simulink model "mainController19a"  (R2019a)
settings: Solver=ode3  StartTime=0  StopTime=inf  FixedStep=0.1  RelTol=1e-3
model workspace (MAT data in the model file):
  SL_ROS_VariableLengthArrays_MaxSizes.CommonInfo.ArrayTruncateAction = 'EmitWarning'
  SL_ROS_VariableLengthArrays_MaxSizes.MsgTypeMap = containers.Map
  SL_ROS_VariableLengthArrays_MaxSizes.MsgTypeMap.serialization.keys = {'sensor_msgs/JointState', 'sensor_msgs/PointCloud2', 'trajectory_msgs/JointTrajectoryPoint'}
  SL_ROS_VariableLengthArrays_MaxSizes.MsgTypeMap.serialization.values{1}(1).PropertyName = 'Name'
  SL_ROS_VariableLengthArrays_MaxSizes.MsgTypeMap.serialization.values{1}(1).DataType = 'std_msgs/String'
  SL_ROS_VariableLengthArrays_MaxSizes.MsgTypeMap.serialization.values{1}(1).MaxLength = 16
  SL_ROS_VariableLengthArrays_MaxSizes.MsgTypeMap.serialization.values{1}(2).PropertyName = 'Position'
  SL_ROS_VariableLengthArrays_MaxSizes.MsgTypeMap.serialization.values{1}(2).DataType = 'double'
  SL_ROS_VariableLengthArrays_MaxSizes.MsgTypeMap.serialization.values{1}(2).MaxLength = 16
  SL_ROS_VariableLengthArrays_MaxSizes.MsgTypeMap.serialization.values{1}(3).PropertyName = 'Velocity'
  SL_ROS_VariableLengthArrays_MaxSizes.MsgTypeMap.serialization.values{1}(3).DataType = 'double'
  SL_ROS_VariableLengthArrays_MaxSizes.MsgTypeMap.serialization.values{1}(3).MaxLength = 16
  SL_ROS_VariableLengthArrays_MaxSizes.MsgTypeMap.serialization.values{1}(4).PropertyName = 'Effort'
  SL_ROS_VariableLengthArrays_MaxSizes.MsgTypeMap.serialization.values{1}(4).DataType = 'double'
  SL_ROS_VariableLengthArrays_MaxSizes.MsgTypeMap.serialization.values{1}(4).MaxLength = 16
  SL_ROS_VariableLengthArrays_MaxSizes.MsgTypeMap.serialization.values{2}(1).PropertyName = 'Data'
  SL_ROS_VariableLengthArrays_MaxSizes.MsgTypeMap.serialization.values{2}(1).DataType = 'uint8'
  SL_ROS_VariableLengthArrays_MaxSizes.MsgTypeMap.serialization.values{2}(1).MaxLength = 9830400
  SL_ROS_VariableLengthArrays_MaxSizes.MsgTypeMap.serialization.values{2}(2).PropertyName = 'Fields'
  SL_ROS_VariableLengthArrays_MaxSizes.MsgTypeMap.serialization.values{2}(2).DataType = 'sensor_msgs/PointField'
  SL_ROS_VariableLengthArrays_MaxSizes.MsgTypeMap.serialization.values{2}(2).MaxLength = 16
  SL_ROS_VariableLengthArrays_MaxSizes.MsgTypeMap.serialization.values{3}(1).PropertyName = 'Positions'
  SL_ROS_VariableLengthArrays_MaxSizes.MsgTypeMap.serialization.values{3}(1).DataType = 'double'
  SL_ROS_VariableLengthArrays_MaxSizes.MsgTypeMap.serialization.values{3}(1).MaxLength = 16
  SL_ROS_VariableLengthArrays_MaxSizes.MsgTypeMap.serialization.values{3}(2).PropertyName = 'Velocities'
  SL_ROS_VariableLengthArrays_MaxSizes.MsgTypeMap.serialization.values{3}(2).DataType = 'double'
  SL_ROS_VariableLengthArrays_MaxSizes.MsgTypeMap.serialization.values{3}(2).MaxLength = 16
  SL_ROS_VariableLengthArrays_MaxSizes.MsgTypeMap.serialization.values{3}(3).PropertyName = 'Accelerations'
  SL_ROS_VariableLengthArrays_MaxSizes.MsgTypeMap.serialization.values{3}(3).DataType = 'double'
  SL_ROS_VariableLengthArrays_MaxSizes.MsgTypeMap.serialization.values{3}(3).MaxLength = 16
  SL_ROS_VariableLengthArrays_MaxSizes.MsgTypeMap.serialization.values{3}(4).PropertyName = 'Effort'
  SL_ROS_VariableLengthArrays_MaxSizes.MsgTypeMap.serialization.values{3}(4).DataType = 'double'
  SL_ROS_VariableLengthArrays_MaxSizes.MsgTypeMap.serialization.values{3}(4).MaxLength = 16
  SL_ROS_VariableLengthArrays_MaxSizes.MsgTypeMap.serialization.uniformity = 0
  SL_ROS_VariableLengthArrays_MaxSizes.MsgTypeMap.serialization.keyType = 'char'
  SL_ROS_VariableLengthArrays_MaxSizes.MsgTypeMap.serialization.valueType = 'any'
values from neighbouring files (symbols this model uses):
  numJoints = MotominiParams.numJoints    [showCompleteDemo.m]
  numPoints = size(Q,2)-2    [showCompleteDemo.m]
undefined symbols (not defined in the file or in its folder): homeToIdleSpline, idleToHomeSpline, Position, Position_SL_Info, Positions, Positions_SL_Info, TimeFromStart, Velocities, Velocities_SL_Info
libraries: robotlib x18, visiontextngfix x3, simulink x2, visionsinks x1
(part 1 of 2)
settings Model: Creator=csantacr  LastModifiedBy=tkikawad
settings DataIOCC: ReturnWorkspaceOutputs=off
settings OptimizationCC: MaxStackSize=64
settings DebuggingCC: ParameterTunabilityLossMsg=error  ArithmeticOperatorsInVariantConditions=warning
settings HardwareCC: ProdBitPerPointer=32  ProdBitPerSizeT=32  ProdBitPerPtrDiffT=32  ProdLargestAtomicFloat=None  ProdIntDivRoundTo=Undefined  ProdEndianess=Unspecified  ProdWordSize=32  ProdHWDeviceType=Generic->Unspecified (assume 32-bit Generic)
settings SFSimCC: SimUseLocalCustomCode=off  MATLABDynamicMemAlloc=off
settings RTWCC: SystemTargetFile=ert.tlc  HardwareBoard=Robot Operating System (ROS)  TLCOptions="-aInlineSetEventsForThisBaseRateFcn=TLC_FALSE -aSuppressMultiTaskScheduler=TLC_FALSE  -aRateBasedStepFcn=0"  TemplateMakefile=ert_default_tmf  GenerateReport=on  RTWUseLocalCustomCode=off  Toolchain=Catkin  IncludeHyperlinkInReport=on  LaunchReport=on  TargetLang=C++  GenerateTraceInfo=on  GenerateTraceReport=on  GenerateTraceReportSl=on  GenerateTraceReportSf=on  GenerateTraceReportEml=on  GenerateWebview=on
settings CodeAppCC: ForceParamTrailComments=on  IgnoreCustomStorageClasses=off  OperatorAnnotations=on  SimulinkDataObjDesc=on  SFDataObjDesc=on  MATLABFcnDesc=on  InsertBlockDesc=on  StateflowObjectComments=on  MATLABSourceComments=on
settings ERTTargetCC: MultiwordLength=2048  SupportVariableSizeSignals=on
settings ConfigComp: CovMetricSettings=dswe
settings SimscapeCC: SimscapeNormalizeSystem=off

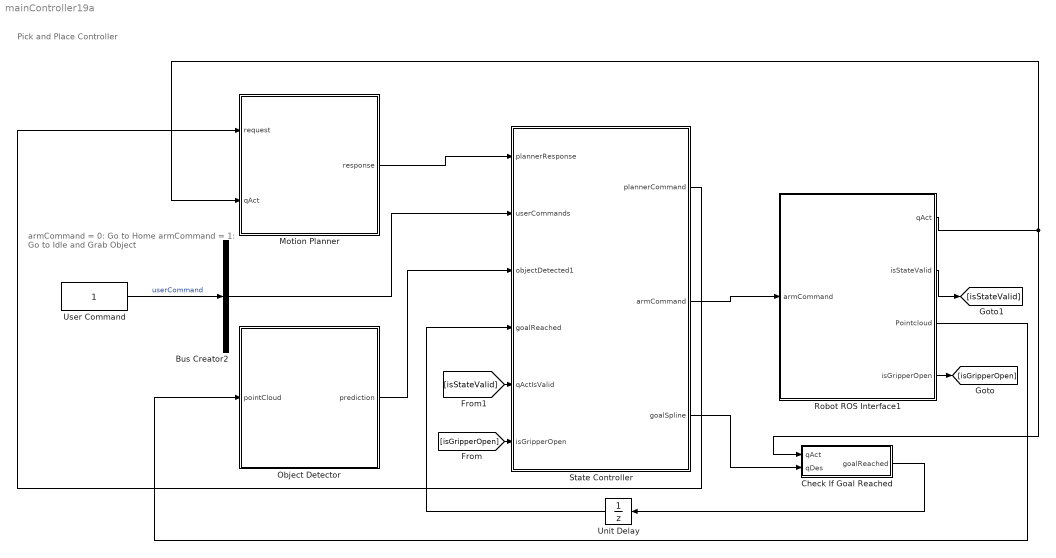
== system mainController19a ==
  note: Pick and Place Controller
  note: armCommand = 0: Go to Home
      | armCommand = 1: Go to Idle and Grab Object
  Bus Creator2 : BusCreator  Inputs=1
  Check If Goal Reached : Subsystem  mask{errorTolerance=50e-3}
      mask prompts: errorTolerance "Error Tolerance"
  Motion Planner : Subsystem
      mask Display: image('youbotMLPlanner.jpg');
  Object Detector : Subsystem
      mask Display: image('clusterFromSML.png');
  Robot ROS Interface1 : Subsystem
  State Controller : Subsystem
  Unit Delay : UnitDelay  SampleTime=-1  HasFrameUpgradeWarning=on
  User Command : Constant  OutDataTypeStr=uint32  SampleTime=0.1
  wires:
  Check If Goal Reached/1(goalReached) -> Unit Delay/1
  User Command/1 -> Bus Creator2/1  "userCommand"
  Robot ROS Interface1/1(qAct) -> Motion Planner/2(qAct), Check If Goal Reached/1(qAct)
  State Controller/3(goalSpline) -> Check If Goal Reached/2(qDes)
  Robot ROS Interface1/2(isStateValid) -> [isStateValid]
  Robot ROS Interface1/3(Pointcloud) -> Object Detector/1(pointCloud)
  Bus Creator2/1 -> State Controller/2(userCommands)
  Motion Planner/1(response) -> State Controller/1(plannerResponse)
  Unit Delay/1 -> State Controller/4(goalReached)
  [isStateValid] -> State Controller/5(qActIsValid)
  State Controller/1(plannerCommand) -> Motion Planner/1(request)
  State Controller/2(armCommand) -> Robot ROS Interface1/1(armCommand)
  Object Detector/1(prediction) -> State Controller/3(objectDetected1)
  Robot ROS Interface1/4(isGripperOpen) -> [isGripperOpen]
  [isGripperOpen] -> State Controller/6(isGripperOpen)

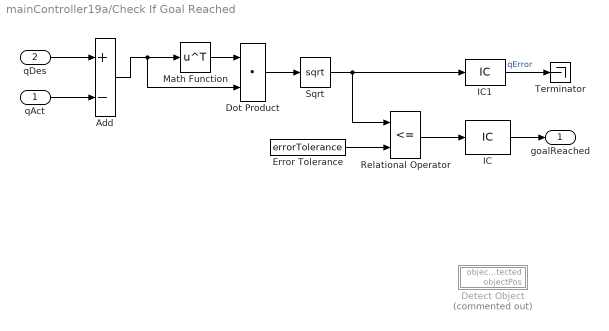
== system mainController19a/Check If Goal Reached ==
  qAct : Inport
  qDes : Inport  Port=2
  Add : Sum  Inputs=+-
  Detect Object : Subsystem  Commented=on
  Dot Product : DotProduct  InputSameDT=on  OutDataTypeStr=Inherit: Inherit via internal rule
  Error Tolerance : Constant  Value=errorTolerance
  IC : InitialCondition  Value=0
  IC1 : InitialCondition  Value=-1000
  Math Function : Math  Operator=transpose  SaturateOnIntegerOverflow=on
  Relational Operator : RelationalOperator  Operator=<=  OutDataTypeStr=boolean  RndMeth=Simplest
  Sqrt : Sqrt  SaturateOnIntegerOverflow=on
  Terminator : Terminator
  goalReached : Outport
  wires:
  Math Function/1 -> Dot Product/1
  Add/1 -> Dot Product/2, Math Function/1
  Dot Product/1 -> Sqrt/1
  qDes/1 -> Add/1
  qAct/1 -> Add/2
  Sqrt/1 -> Relational Operator/1, IC1/1
  Relational Operator/1 -> IC/1
  Error Tolerance/1 -> Relational Operator/2
  IC/1 -> goalReached/1
  IC1/1 -> Terminator/1  "qError"

== system mainController19a/Motion Planner ==
  request : Inport
  qAct : Inport  Port=2
  Bus Creator : BusCreator  Inputs=5
  Bus Selector : BusSelector  OutputSignals=plannerRequest,plannerPos,plannerID
  Planner Response : Subsystem
  Request Motion Plan : Subsystem  TreatAsAtomicUnit=on
  response : Outport
  wires:
  Planner Response/4(t) -> Bus Creator/4
  request/1 -> Bus Selector/1
  Planner Response/3(dQ) -> Bus Creator/3
  Planner Response/2(Q) -> Bus Creator/2
  Planner Response/5(isValid) -> Bus Creator/5
  Planner Response/1(hasData) -> Bus Creator/1
  Bus Selector/2 -> Request Motion Plan/1(objectPos)  "<plannerPos>"
  Bus Creator/1 -> response/1
  qAct/1 -> Request Motion Plan/3(qAct)
  Bus Selector/1 -> Request Motion Plan/Trigger  "<plannerRequest>"
  Bus Selector/3 -> Request Motion Plan/2(objectID)  "<plannerID>"

== system mainController19a/Object Detector ==
  pointCloud : Inport
  Bus Creator : BusCreator  Inputs=2
  Bus Selector : BusSelector  OutputSignals=RGB,XYZ
  Data Type Conversion1 : DataTypeConversion  OutDataTypeStr=uint32
  Display : Subsystem
  ObjectDetector : MATLABSystem  System=ObjectDetector  roi=[ 20, 240, 600, 240 ]  tform=b_T_k  SimulateUsing=Interpreted execution
      mask Type: ObjectDetector
      mask Display:
      | disp('ObjectDetector');
      | port_label('input',1,'im');
      | port_label('input',2,'pts');
      | port_label('output',1,'predictedLabels');
      | port_label('output',2,'bboxes');
      | port_label('output',3,'xyzPoints');
  prediction : Outport
  wires:
  Bus Selector/1 -> ObjectDetector/1, Display/1(Image)  "<RGB>"
  ObjectDetector/2 -> Display/3(bboxes)
  Bus Selector/2 -> ObjectDetector/2  "<XYZ>"
  ObjectDetector/1 -> Data Type Conversion1/1, Display/2(Labels)
  ObjectDetector/3 -> Bus Creator/2, Display/4(xyzPoints)  "xyzPoints"
  pointCloud/1 -> Bus Selector/1
  Bus Creator/1 -> prediction/1
  Data Type Conversion1/1 -> Bus Creator/1  "predictedLabels"

== system mainController19a/Robot ROS Interface1 ==
  armCommand : Inport
  Arm Trajectory Controller : Subsystem  mask{numJoints=numJoints}
      mask prompts: numJoints "Number of Joints"
      mask Display: %image('rosorg-logo.png',[0.25 0.35 0.5 0.3]);
  Bus Creator : BusCreator  Inputs=2
  Bus Selector : BusSelector  OutputSignals=requestTrajController,Qspline,dQspline,tSpline,requestGripController,gripCommand
  Display : Display
  Gripper Trajectory Controller : Subsystem  mask{numJoints=2}
      mask prompts: numJoints "Number of Joints"
      mask Display: %image('rosorg-logo.png',[0.25 0.35 0.5 0.3]);
  Kinect Data : Subsystem
  Robot State : Subsystem  mask{numJoints=numJoints}
      mask prompts: numJoints "Number of Joints"
      mask Display: %image('rosorg-logo.png',[0.25 0.35 0.5 0.3]);
  qAct : Outport
  isStateValid : Outport  Port=2
  Pointcloud : Outport  Port=3
  isGripperOpen : Outport  Port=4
  wires:
  Bus Selector/6 -> Gripper Trajectory Controller/1(gripperCmd)  "<gripCommand>"
  Robot State/3(isGripperOpen) -> isGripperOpen/1
  Robot State/2(qAct) -> qAct/1
  Bus Selector/2 -> Display/1, Arm Trajectory Controller/1(qMatrix)  "<Qspline>"
  Bus Selector/3 -> Arm Trajectory Controller/2(dqMatrix)  "<dQspline>"
  Robot State/1(isValid) -> isStateValid/1
  armCommand/1 -> Bus Selector/1
  Bus Selector/4 -> Arm Trajectory Controller/3(tVector)  "<tSpline>"
  Bus Selector/5 -> Gripper Trajectory Controller/Trigger  "<requestGripController>"
  Kinect Data/1(RGB) -> Bus Creator/1  "RGB"
  Kinect Data/2(XYZ) -> Bus Creator/2  "XYZ"
  Bus Creator/1 -> Pointcloud/1
  Bus Selector/1 -> Arm Trajectory Controller/Trigger  "<requestTrajController>"

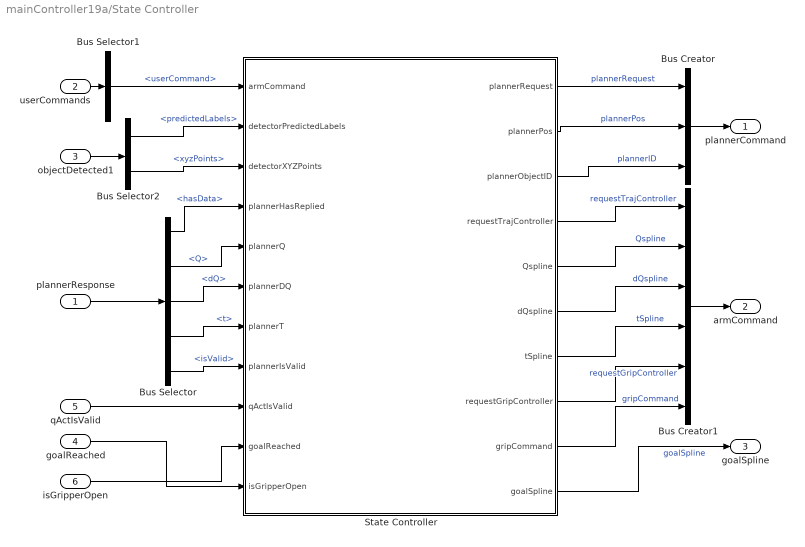
== system mainController19a/State Controller ==
  plannerResponse : Inport
  userCommands : Inport  Port=2
  objectDetected1 : Inport  Port=3
  goalReached : Inport  Port=4
  qActIsValid : Inport  Port=5
  isGripperOpen : Inport  Port=6
  Bus Creator : BusCreator  Inputs=3
  Bus Creator1 : BusCreator  Inputs=6
  Bus Selector : BusSelector  OutputSignals=hasData,Q,dQ,t,isValid
  Bus Selector1 : BusSelector  OutputSignals=userCommand
  Bus Selector2 : BusSelector  OutputSignals=predictedLabels,xyzPoints
  State Controller : Stateflow chart  TreatAsAtomicUnit=on
  plannerCommand : Outport
  armCommand : Outport  Port=2
  goalSpline : Outport  Port=3
  wires:
  Bus Creator/1 -> plannerCommand/1
  qActIsValid/1 -> State Controller/9(qActIsValid)
  Bus Creator1/1 -> armCommand/1
  goalReached/1 -> State Controller/11(isGripperOpen)
  State Controller/10(goalSpline) -> goalSpline/1  "goalSpline"
  Bus Selector1/1 -> State Controller/1(armCommand)  "<userCommand>"
  userCommands/1 -> Bus Selector1/1
  State Controller/9(gripCommand) -> Bus Creator1/6  "gripCommand"
  State Controller/8(requestGripController) -> Bus Creator1/5  "requestGripController"
  State Controller/5(Qspline) -> Bus Creator1/2  "Qspline"
  State Controller/4(requestTrajController) -> Bus Creator1/1  "requestTrajController"
  State Controller/6(dQspline) -> Bus Creator1/3  "dQspline"
  State Controller/7(tSpline) -> Bus Creator1/4  "tSpline"
  Bus Selector/1 -> State Controller/4(plannerHasReplied)  "<hasData>"
  Bus Selector/3 -> State Controller/6(plannerDQ)  "<dQ>"
  State Controller/2(plannerPos) -> Bus Creator/2  "plannerPos"
  plannerResponse/1 -> Bus Selector/1
  Bus Selector/2 -> State Controller/5(plannerQ)  "<Q>"
  State Controller/1(plannerRequest) -> Bus Creator/1  "plannerRequest"
  Bus Selector/4 -> State Controller/7(plannerT)  "<t>"
  State Controller/3(plannerObjectID) -> Bus Creator/3  "plannerID"
  Bus Selector/5 -> State Controller/8(plannerIsValid)  "<isValid>"
  objectDetected1/1 -> Bus Selector2/1
  Bus Selector2/1 -> State Controller/2(detectorPredictedLabels)  "<predictedLabels>"
  Bus Selector2/2 -> State Controller/3(detectorXYZPoints)  "<xyzPoints>"
  isGripperOpen/1 -> State Controller/10(goalReached)

== system mainController19a/Check If Goal Reached/Detect Object ==
  note: 1:Blue
      | 2:Turquoise
      | 3:Purple
  Manual Switch : ManualSwitch
  Manual Switch1 : ManualSwitch
  Manual Switch2 : ManualSwitch  CurrentSetting=0
  Manual Switch3 : ManualSwitch
  object Detected : Constant  OutDataTypeStr=uint32
  object Detected Pos : Constant  Value=[0.28 0.12 0.0]  OutDataTypeStr=double
  object Detected Pos1 : Constant  Value=[0.28 0.0 0.0]  OutDataTypeStr=double
  object Detected Pos2 : Constant  Value=[0.28 -0.12 0.0]  OutDataTypeStr=double
  object Detected1 : Constant  Value=2  OutDataTypeStr=uint32
  object Detected2 : Constant  Value=3  OutDataTypeStr=uint32
  objectDetected : Outport
  objectPos : Outport  Port=2
  wires:
  object Detected Pos/1 -> Manual Switch2/1
  object Detected/1 -> Manual Switch/1
  object Detected1/1 -> Manual Switch/2
  Manual Switch/1 -> Manual Switch1/1
  Manual Switch1/1 -> objectDetected/1
  object Detected2/1 -> Manual Switch1/2
  Manual Switch2/1 -> Manual Switch3/1
  Manual Switch3/1 -> objectPos/1
  object Detected Pos1/1 -> Manual Switch2/2
  object Detected Pos2/1 -> Manual Switch3/2

== system mainController19a/Motion Planner/Planner Response ==
  Joint Trajectory to Spline Matrices : Subsystem  TreatAsAtomicUnit=on  mask{numJoints=numJoints, numPoints=numPoints}
      mask prompts: numJoints "Number of Joints"; numPoints "Number of Points"
  Subscribe : robotlib/Subscribe  topicSource=Specify your own  topic=/planner/joint_trajectory  messageType=trajectory_msgs/JointTrajectory  sampleTime=-1  messageQueueLength=1
      settings: SourceProductBaseCode=RO
  hasData : Outport
  Q : Outport  Port=2
  dQ : Outport  Port=3
  t : Outport  Port=4
  isValid : Outport  Port=5
  wires:
  Subscribe/2 -> Joint Trajectory to Spline Matrices/1(jntTrajMsg)
  Joint Trajectory to Spline Matrices/1(Q) -> Q/1  "Q"
  Joint Trajectory to Spline Matrices/2(dQ) -> dQ/1  "dQ"
  Joint Trajectory to Spline Matrices/3(t) -> t/1  "t"
  Subscribe/1 -> Joint Trajectory to Spline Matrices/Trigger, hasData/1  "hasData"
  Joint Trajectory to Spline Matrices/4(isValid) -> isValid/1  "isValid"

== system mainController19a/Motion Planner/Request Motion Plan ==
  objectPos : Inport
  objectID : Inport  Port=2
  qAct : Inport  Port=3
  Trigger : TriggerPort  VariantControl=Variant  PortDimensions=1
  Assignment : Assignment  DiagnosticForDimensions=Warning  IndexOptions=Index vector (dialog)  Indices=1:numJoints+4  OutputSizes=1
  Blank Message1 : robotlib/Blank Message  messageClass=Message  entityType=sensor_msgs/JointState  messageType=sensor_msgs/JointState  SampleTime=-1
      settings: SourceProductBaseCode=RO
  Bus Assignment1 : BusAssignment  AssignedSignals=Position,Position_SL_Info.CurrentLength
  Constant : Constant  Value=zeros(16,1)
  Data Type Conversion : DataTypeConversion  OutDataTypeStr=double
  Data Type Conversion1 : DataTypeConversion  OutDataTypeStr=uint32
  Publish1 : robotlib/Publish  topicSource=Specify your own  topic=/planner/request  messageType=sensor_msgs/JointState  messageQueueLength=1
      settings: SourceProductBaseCode=RO
  Vector Concatenate : Concatenate  NumInputs=3
  Width : Width
  wires:
  objectPos/1 -> Vector Concatenate/1
  objectID/1 -> Data Type Conversion/1
  Data Type Conversion/1 -> Vector Concatenate/2
  Blank Message1/1 -> Bus Assignment1/1
  Bus Assignment1/1 -> Publish1/1
  qAct/1 -> Vector Concatenate/3
  Vector Concatenate/1 -> Width/1, Assignment/2
  Assignment/1 -> Bus Assignment1/2
  Constant/1 -> Assignment/1
  Width/1 -> Data Type Conversion1/1
  Data Type Conversion1/1 -> Bus Assignment1/3

== system mainController19a/Object Detector/Display ==
  Image : Inport
  Labels : Inport  Port=2
  bboxes : Inport  Port=3
  xyzPoints : Inport  Port=4
  Data Type Conversion : DataTypeConversion  OutDataTypeStr=int32
  Data Type Conversion1 : DataTypeConversion  OutDataTypeStr=single
  Draw Shapes : visiontextngfix/Draw Shapes  shape=Rectangles  fill=off  lineWidth=3  fillClrSource=Specify via dialog  display=User-specified value  intensity=200  color=[1 0 0]  opacity=0.6  viewport=Entire image  antialiasing=off  inType=Obsolete  imagePorts=One multidimensional signal  roundingMode=Floor  overflowMode=off  memoryMode=Specify word length  memoryWordLength=16  prodOutputMode=Binary point scaling  prodOutputWordLength=32  prodOutputFracLength=14  prodOutputSlope=2^-14  accumSlope=2^-14  memoryFracLength=15
      settings: SourceProductName=Computer Vision Toolbox
  Formatting : MATLAB Function  TreatAsAtomicUnit=on
  Insert Text : visiontextngfix/Insert Text  inputType=Obsolete  theText='%d'  getTextLocFrom=Input port  textLoc=[1 1]  getTextColorFrom=Specify via dialog  textColor=[1 0 0]  getTextIntensityFrom=Specify via dialog  textIntensity=0  getTextOpacityFrom=Specify via dialog  textOpacity=1.0  dummyVar2=0  dummyVar3=0  dummyVar4=0  imagePorts=One multidimensional signal  isInputTransposed=off  fontFace=LucidaSansRegular  dummyVar1=0  blockFontSize=30  antiAliased=on
      settings: SourceProductName=Computer Vision Toolbox  SourceProductBaseCode=VP
  Insert Text1 : visiontextngfix/Insert Text  inputType=Obsolete  theText='#%1.0f, Label:%1.0f, X:% 2.2f, Y:% 2.2f, Z:% 2.2f'  getTextLocFrom=Input port  textLoc=[1 1]  getTextColorFrom=Input port  textColor=[1 0 0]  getTextIntensityFrom=Specify via dialog  textIntensity=0  getTextOpacityFrom=Specify via dialog  textOpacity=1.0  dummyVar2=0  dummyVar3=0  dummyVar4=0  imagePorts=One multidimensional signal  isInputTransposed=off  fontFace=LucidaSansRegular  dummyVar1=0  blockFontSize=30  antiAliased=on
      settings: SourceProductName=Computer Vision Toolbox  SourceProductBaseCode=VP
  MATLAB Function : MATLAB Function  TreatAsAtomicUnit=on
  Select Top-left points : Selector  NumberOfDimensions=2  InputPortWidth=3  IndexOptions=Select all,Index vector (dialog)  Indices=[1 3],1:2  OutputSizes=1,1
  To Video Display1 : visionsinks/To Video Display  windowSizeMode=Normal  openAtMdlStart=on  fullScreen=off  videoWindowX=36  videoWindowY=413  saveWindowSize=off  videoWindowWidth=332  videoWindowHeight=283  inputColorFormat=RGB  inputType=Obsolete  imagePorts=One multidimensional signal  OutputDevice=On-screen video monitor  dataOrg=Column-major  isWindowOpen=off
      settings: SourceProductName=Computer Vision Toolbox
  wires:
  Formatting/1(Variables) -> Insert Text1/2
  Formatting/3(Location) -> Insert Text1/4
  Labels/1 -> Formatting/1(predictedLabels), MATLAB Function/1(u)
  Formatting/2(Color) -> Insert Text1/3
  xyzPoints/1 -> Formatting/2(xyzPoints)
  Image/1 -> Data Type Conversion1/1
  MATLAB Function/1(y) -> Insert Text/2
  Insert Text/1 -> Insert Text1/1
  bboxes/1 -> Draw Shapes/2, Select Top-left points/1
  Insert Text1/1 -> To Video Display1/1
  Select Top-left points/1 -> Data Type Conversion/1
  Draw Shapes/1 -> Insert Text/1
  Data Type Conversion/1 -> Insert Text/3
  Data Type Conversion1/1 -> Draw Shapes/1

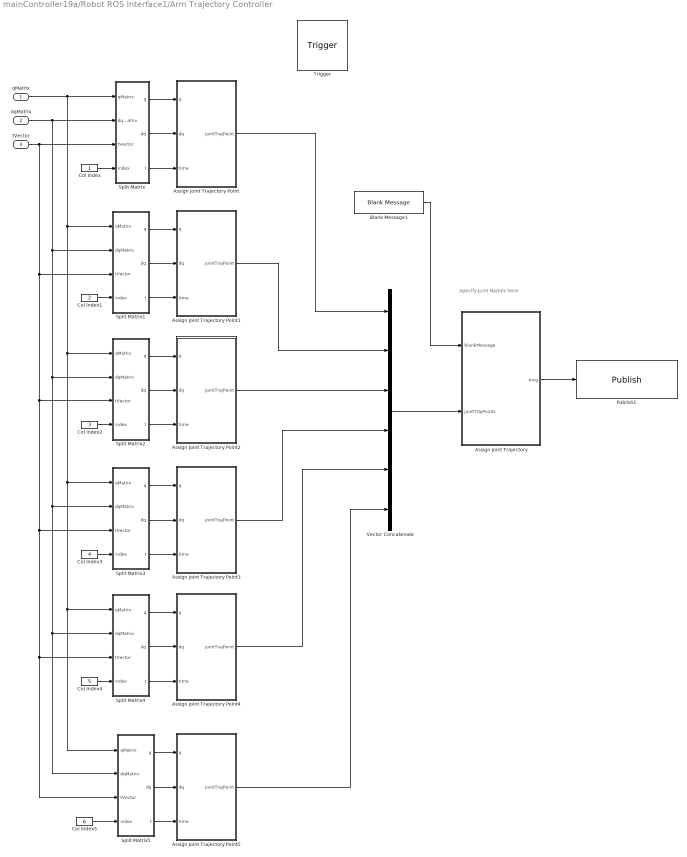
== system mainController19a/Robot ROS Interface1/Arm Trajectory Controller ==
  note: Specify Joint Names here
  qMatrix : Inport
  dqMatrix : Inport  Port=2
  tVector : Inport  Port=3
  Trigger : TriggerPort  VariantControl=Variant  PortDimensions=1
  " Assign Joint Trajectory" : MATLAB Function  TreatAsAtomicUnit=on
  Assign Joint Trajectory Point : Subsystem  mask{numJoints=numJoints}
      mask prompts: numJoints "Number of Joints"
  Assign Joint Trajectory Point1 : Subsystem  mask{numJoints=numJoints}
      mask prompts: numJoints "Number of Joints"
  Assign Joint Trajectory Point2 : Subsystem  mask{numJoints=numJoints}
      mask prompts: numJoints "Number of Joints"
  Assign Joint Trajectory Point3 : Subsystem  mask{numJoints=numJoints}
      mask prompts: numJoints "Number of Joints"
  Assign Joint Trajectory Point4 : Subsystem  mask{numJoints=numJoints}
      mask prompts: numJoints "Number of Joints"
  Assign Joint Trajectory Point5 : Subsystem  mask{numJoints=numJoints}
      mask prompts: numJoints "Number of Joints"
  Blank Message1 : robotlib/Blank Message  messageClass=Message  entityType=trajectory_msgs/JointTrajectory  messageType=trajectory_msgs/JointTrajectory  SampleTime=-1
      settings: SourceProductBaseCode=RO
  Col Index : Constant
  Col Index1 : Constant  Value=2
  Col Index2 : Constant  Value=3
  Col Index3 : Constant  Value=4
  Col Index4 : Constant  Value=5
  Col Index5 : Constant  Value=6
  Publish1 : robotlib/Publish  topicSource=Select from ROS network  topic=/motomini_controller/command  messageType=trajectory_msgs/JointTrajectory  messageQueueLength=1
      settings: SourceProductBaseCode=RO
  Split Matrix : Subsystem
  Split Matrix1 : Subsystem
  Split Matrix2 : Subsystem
  Split Matrix3 : Subsystem
  Split Matrix4 : Subsystem
  Split Matrix5 : Subsystem
  Vector Concatenate : Concatenate  NumInputs=6
  wires:
  Assign Joint Trajectory Point/1(jointTrajPoint) -> Vector Concatenate/1
  Assign Joint Trajectory Point1/1(jointTrajPoint) -> Vector Concatenate/2
  Vector Concatenate/1 -> " Assign Joint Trajectory"/2(jointTrajPoints)
  Blank Message1/1 -> " Assign Joint Trajectory"/1(blankMessage)
  " Assign Joint Trajectory"/1(msg) -> Publish1/1
  qMatrix/1 -> Split Matrix5/1(qMatrix), Split Matrix4/1(qMatrix), Split Matrix3/1(qMatrix), Split Matrix2/1(qMatrix), Split Matrix1/1(qMatrix), Split Matrix/1(qMatrix)
  Assign Joint Trajectory Point2/1(jointTrajPoint) -> Vector Concatenate/3
  tVector/1 -> Split Matrix2/3(tVector), Split Matrix3/3(tVector), Split Matrix5/3(tVector), Split Matrix4/3(tVector), Split Matrix1/3(tVector), Split Matrix/3(tVector)
  Col Index/1 -> Split Matrix/4(index)
  Split Matrix/1(q) -> Assign Joint Trajectory Point/1(q)
  Split Matrix/2(dq) -> Assign Joint Trajectory Point/2(dq)
  Split Matrix/3(t) -> Assign Joint Trajectory Point/3(time)
  Split Matrix1/1(q) -> Assign Joint Trajectory Point1/1(q)
  Split Matrix1/2(dq) -> Assign Joint Trajectory Point1/2(dq)
  Split Matrix1/3(t) -> Assign Joint Trajectory Point1/3(time)
  Split Matrix2/1(q) -> Assign Joint Trajectory Point2/1(q)
  Split Matrix2/3(t) -> Assign Joint Trajectory Point2/3(time)
  Split Matrix2/2(dq) -> Assign Joint Trajectory Point2/2(dq)
  Split Matrix3/3(t) -> Assign Joint Trajectory Point3/3(time)
  Split Matrix4/3(t) -> Assign Joint Trajectory Point4/3(time)
  Assign Joint Trajectory Point3/1(jointTrajPoint) -> Vector Concatenate/4
  Assign Joint Trajectory Point4/1(jointTrajPoint) -> Vector Concatenate/5
  dqMatrix/1 -> Split Matrix2/2(dqMatrix), Split Matrix3/2(dqMatrix), Split Matrix4/2(dqMatrix), Split Matrix5/2(dqMatrix), Split Matrix1/2(dqMatrix), Split Matrix/2(dqMatrix)
  Split Matrix3/1(q) -> Assign Joint Trajectory Point3/1(q)
  Split Matrix3/2(dq) -> Assign Joint Trajectory Point3/2(dq)
  Split Matrix4/2(dq) -> Assign Joint Trajectory Point4/2(dq)
  Split Matrix4/1(q) -> Assign Joint Trajectory Point4/1(q)
  Col Index1/1 -> Split Matrix1/4(index)
  Col Index2/1 -> Split Matrix2/4(index)
  Col Index3/1 -> Split Matrix3/4(index)
  Col Index4/1 -> Split Matrix4/4(index)
  Split Matrix5/1(q) -> Assign Joint Trajectory Point5/1(q)
  Split Matrix5/2(dq) -> Assign Joint Trajectory Point5/2(dq)
  Split Matrix5/3(t) -> Assign Joint Trajectory Point5/3(time)
  Col Index5/1 -> Split Matrix5/4(index)
  Assign Joint Trajectory Point5/1(jointTrajPoint) -> Vector Concatenate/6

== system mainController19a/Robot ROS Interface1/Gripper Trajectory Controller ==
  note: Specify Joint Names here
  gripperCmd : Inport
  Trigger : TriggerPort  VariantControl=Variant  PortDimensions=1
  " Assign Joint Trajectory" : MATLAB Function  TreatAsAtomicUnit=on
  Assign Joint Trajectory Point : Subsystem  mask{numJoints=2}
      mask prompts: numJoints "Number of Joints"
  Blank Message1 : robotlib/Blank Message  messageClass=Message  entityType=trajectory_msgs/JointTrajectory  messageType=trajectory_msgs/JointTrajectory  SampleTime=-1
      settings: SourceProductBaseCode=RO
  Constant : Constant  Value=[0;0]
  Constant1 : Constant  Value=2
  Publish1 : robotlib/Publish  topicSource=Select from ROS network  topic=/gripper_controller/command  messageType=trajectory_msgs/JointTrajectory  messageQueueLength=1
      settings: SourceProductBaseCode=RO
  Vector Concatenate : Concatenate  NumInputs=1
  wires:
  Constant1/1 -> Assign Joint Trajectory Point/3(time)
  Constant/1 -> Assign Joint Trajectory Point/2(dq)
  gripperCmd/1 -> Assign Joint Trajectory Point/1(q)
  " Assign Joint Trajectory"/1(msg) -> Publish1/1
  Blank Message1/1 -> " Assign Joint Trajectory"/1(blankMessage)
  Vector Concatenate/1 -> " Assign Joint Trajectory"/2(jointTrajPoints)
  Assign Joint Trajectory Point/1(jointTrajPoint) -> Vector Concatenate/1

== system mainController19a/Robot ROS Interface1/Kinect Data ==
  Extract Point Cloud Data : Subsystem  TreatAsAtomicUnit=on
  Subscribe : robotlib/Subscribe  topicSource=Select from ROS network  topic=/kinect2/sd/points  messageType=sensor_msgs/PointCloud2  sampleTime=1  messageQueueLength=1
      settings: SourceProductBaseCode=RO
  RGB : Outport
  XYZ : Outport  Port=2
  wires:
  Subscribe/2 -> Extract Point Cloud Data/1(pcloudMsg)
  Subscribe/1 -> Extract Point Cloud Data/Enable
  Extract Point Cloud Data/2(XYZ) -> XYZ/1
  Extract Point Cloud Data/1(RGB) -> RGB/1

== system mainController19a/Robot ROS Interface1/Robot State ==
  Compare To Constant : simulink/Logic and Bit Operations/Compare To Constant  relop=>  const=0.02  OutDataTypeStr=boolean
  Compare To Constant1 : simulink/Logic and Bit Operations/Compare To Constant  relop=>  const=0.02  OutDataTypeStr=boolean
  Demux : Demux  Outputs=2
  Get Finger Positions : Subsystem  mask{numJoints=2}
      mask prompts: numJoints "Number of Joints"
  Get Joint Positions : Subsystem  mask{numJoints=numJoints}
      mask prompts: numJoints "Number of Joints"
  Logical Operator : Logic  AllPortsSameDT=off  OutDataTypeStr=boolean
  Logical Operator1 : Logic  AllPortsSameDT=off  OutDataTypeStr=boolean
  Subscribe : robotlib/Subscribe  topicSource=Select from ROS network  topic=/motomini_controller/state  messageType=control_msgs/JointTrajectoryControllerState  sampleTime=-1  messageQueueLength=1
      settings: SourceProductBaseCode=RO
  Subscribe1 : robotlib/Subscribe  topicSource=Select from ROS network  topic=/gripper_controller/state  messageType=control_msgs/JointTrajectoryControllerState  sampleTime=-1  messageQueueLength=1
      settings: SourceProductBaseCode=RO
  isValid : Outport
  qAct : Outport  Port=2
  isGripperOpen : Outport  Port=3
  wires:
  Get Joint Positions/2(isValid) -> Logical Operator/1
  Subscribe/1 -> Get Joint Positions/Enable
  Subscribe/2 -> Get Joint Positions/1(msg)
  Get Joint Positions/1(qAct) -> qAct/1
  Subscribe1/2 -> Get Finger Positions/1(msg)
  Subscribe1/1 -> Get Finger Positions/Enable
  Get Finger Positions/1(gripperAct) -> Demux/1
  Get Finger Positions/2(isValid) -> Logical Operator/2
  Logical Operator/1 -> isValid/1
  Demux/1 -> Compare To Constant/1
  Demux/2 -> Compare To Constant1/1
  Compare To Constant/1 -> Logical Operator1/1
  Compare To Constant1/1 -> Logical Operator1/2
  Logical Operator1/1 -> isGripperOpen/1

== system mainController19a/Motion Planner/Planner Response/Joint Trajectory to Spline Matrices ==
  jntTrajMsg : Inport
  Trigger : TriggerPort  VariantControl=Variant
  Bus Selector : BusSelector  OutputSignals=Points,Points_SL_Info.CurrentLength
  Constant : Constant  Value=numPoints+2
  Data Type Conversion : DataTypeConversion  OutDataTypeStr=uint32
  Logical Operator : Logic  AllPortsSameDT=off  OutDataTypeStr=boolean
  Relational Operator : RelationalOperator  Operator===  OutDataTypeStr=boolean  RndMeth=Simplest
  pointsToSplineData : MATLAB Function  TreatAsAtomicUnit=on  mask{numJoints=numJoints, numPoints=numPoints}
      mask prompts: numJoints "Number of Joints"; numPoints "Number of Points"
  pointsToSplineWithBlocks : Subsystem  Commented=on
  Q : Outport  InitialOutput=zeros(numJoints, numPoints+2)
  dQ : Outport  Port=2  InitialOutput=zeros(numJoints, numPoints+2)
  t : Outport  Port=3  InitialOutput=zeros(1, numPoints+2)
  isValid : Outport  Port=4  InitialOutput=[false]
  wires:
  jntTrajMsg/1 -> Bus Selector/1
  Bus Selector/2 -> Relational Operator/1  "<CurrentLength>"
  pointsToSplineData/1(Q) -> Q/1
  pointsToSplineData/2(dQ) -> dQ/1
  pointsToSplineData/3(t) -> t/1
  Bus Selector/1 -> pointsToSplineData/1(pointsMsg)  "<Points>"
  pointsToSplineData/4(isValid) -> Logical Operator/1
  Constant/1 -> Data Type Conversion/1
  Data Type Conversion/1 -> Relational Operator/2
  Relational Operator/1 -> Logical Operator/2
  Logical Operator/1 -> isValid/1

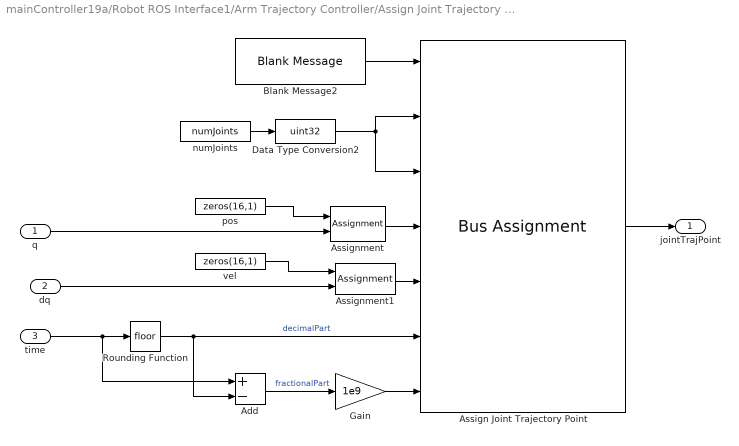
== system mainController19a/Robot ROS Interface1/Arm Trajectory Controller/Assign Joint Trajectory Point ==
  q : Inport
  dq : Inport  Port=2
  time : Inport  Port=3
  Add : Sum  Inputs=+-
  Assign Joint Trajectory Point : BusAssignment  AssignedSignals=Positions_SL_Info.CurrentLength,Velocities_SL_Info.CurrentLength,Positions,Velocities,TimeFromStart.Sec,TimeFromStart.Nsec
  Assignment : Assignment  DiagnosticForDimensions=Warning  IndexOptions=Index vector (dialog)  Indices=1:numJoints  OutputSizes=1
  Assignment1 : Assignment  DiagnosticForDimensions=Warning  IndexOptions=Index vector (dialog)  Indices=1:numJoints  OutputSizes=1
  Blank Message2 : robotlib/Blank Message  messageClass=Message  entityType=trajectory_msgs/JointTrajectoryPoint  messageType=trajectory_msgs/JointTrajectoryPoint  SampleTime=-1
      settings: SourceProductBaseCode=RO
  Data Type Conversion2 : DataTypeConversion  OutDataTypeStr=uint32
  Gain : Gain  Gain=1e9
  Rounding Function : Rounding
  numJoints : Constant  Value=numJoints
  pos : Constant  Value=zeros(16,1)
  vel : Constant  Value=zeros(16,1)
  jointTrajPoint : Outport
  wires:
  Assignment/1 -> Assign Joint Trajectory Point/4
  Assign Joint Trajectory Point/1 -> jointTrajPoint/1
  pos/1 -> Assignment/1
  Gain/1 -> Assign Joint Trajectory Point/7
  q/1 -> Assignment/2
  numJoints/1 -> Data Type Conversion2/1
  Data Type Conversion2/1 -> Assign Joint Trajectory Point/3, Assign Joint Trajectory Point/2
  dq/1 -> Assignment1/2
  Blank Message2/1 -> Assign Joint Trajectory Point/1
  vel/1 -> Assignment1/1
  Assignment1/1 -> Assign Joint Trajectory Point/5
  time/1 -> Add/1, Rounding Function/1
  Rounding Function/1 -> Assign Joint Trajectory Point/6, Add/2  "decimalPart"
  Add/1 -> Gain/1  "fractionalPart"

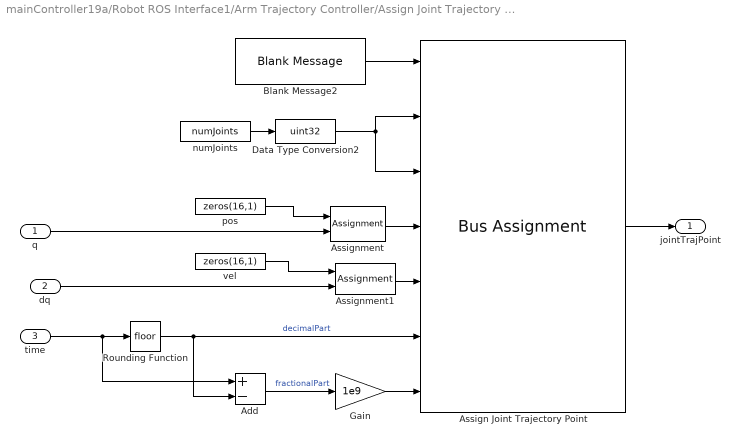
== system mainController19a/Robot ROS Interface1/Arm Trajectory Controller/Assign Joint Trajectory Point1 ==
  q : Inport
  dq : Inport  Port=2
  time : Inport  Port=3
  Add : Sum  Inputs=+-
  Assign Joint Trajectory Point : BusAssignment  AssignedSignals=Positions_SL_Info.CurrentLength,Velocities_SL_Info.CurrentLength,Positions,Velocities,TimeFromStart.Sec,TimeFromStart.Nsec
  Assignment : Assignment  DiagnosticForDimensions=Warning  IndexOptions=Index vector (dialog)  Indices=1:numJoints  OutputSizes=1
  Assignment1 : Assignment  DiagnosticForDimensions=Warning  IndexOptions=Index vector (dialog)  Indices=1:numJoints  OutputSizes=1
  Blank Message2 : robotlib/Blank Message  messageClass=Message  entityType=trajectory_msgs/JointTrajectoryPoint  messageType=trajectory_msgs/JointTrajectoryPoint  SampleTime=-1
      settings: SourceProductBaseCode=RO
  Data Type Conversion2 : DataTypeConversion  OutDataTypeStr=uint32
  Gain : Gain  Gain=1e9
  Rounding Function : Rounding
  numJoints : Constant  Value=numJoints
  pos : Constant  Value=zeros(16,1)
  vel : Constant  Value=zeros(16,1)
  jointTrajPoint : Outport
  wires:
  Add/1 -> Gain/1  "fractionalPart"
  Rounding Function/1 -> Add/2, Assign Joint Trajectory Point/6  "decimalPart"
  time/1 -> Rounding Function/1, Add/1
  Assignment1/1 -> Assign Joint Trajectory Point/5
  vel/1 -> Assignment1/1
  Blank Message2/1 -> Assign Joint Trajectory Point/1
  dq/1 -> Assignment1/2
  Data Type Conversion2/1 -> Assign Joint Trajectory Point/2, Assign Joint Trajectory Point/3
  numJoints/1 -> Data Type Conversion2/1
  q/1 -> Assignment/2
  Gain/1 -> Assign Joint Trajectory Point/7
  pos/1 -> Assignment/1
  Assign Joint Trajectory Point/1 -> jointTrajPoint/1
  Assignment/1 -> Assign Joint Trajectory Point/4

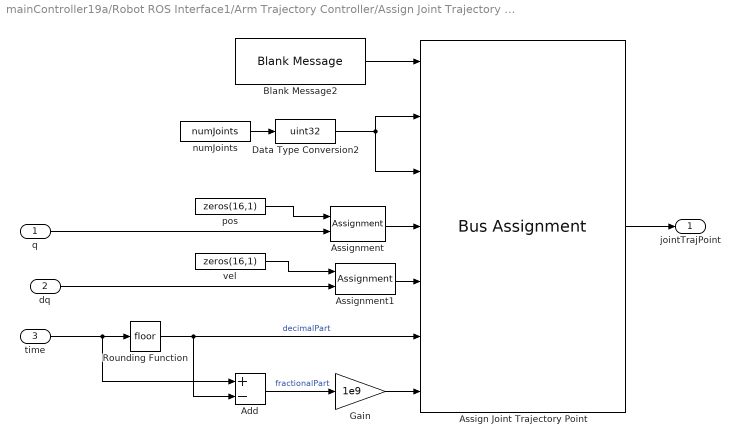
== system mainController19a/Robot ROS Interface1/Arm Trajectory Controller/Assign Joint Trajectory Point2 ==
  q : Inport
  dq : Inport  Port=2
  time : Inport  Port=3
  Add : Sum  Inputs=+-
  Assign Joint Trajectory Point : BusAssignment  AssignedSignals=Positions_SL_Info.CurrentLength,Velocities_SL_Info.CurrentLength,Positions,Velocities,TimeFromStart.Sec,TimeFromStart.Nsec
  Assignment : Assignment  DiagnosticForDimensions=Warning  IndexOptions=Index vector (dialog)  Indices=1:numJoints  OutputSizes=1
  Assignment1 : Assignment  DiagnosticForDimensions=Warning  IndexOptions=Index vector (dialog)  Indices=1:numJoints  OutputSizes=1
  Blank Message2 : robotlib/Blank Message  messageClass=Message  entityType=trajectory_msgs/JointTrajectoryPoint  messageType=trajectory_msgs/JointTrajectoryPoint  SampleTime=-1
      settings: SourceProductBaseCode=RO
  Data Type Conversion2 : DataTypeConversion  OutDataTypeStr=uint32
  Gain : Gain  Gain=1e9
  Rounding Function : Rounding
  numJoints : Constant  Value=numJoints
  pos : Constant  Value=zeros(16,1)
  vel : Constant  Value=zeros(16,1)
  jointTrajPoint : Outport
  wires:
  Assignment/1 -> Assign Joint Trajectory Point/4
  Assign Joint Trajectory Point/1 -> jointTrajPoint/1
  pos/1 -> Assignment/1
  Gain/1 -> Assign Joint Trajectory Point/7
  q/1 -> Assignment/2
  numJoints/1 -> Data Type Conversion2/1
  Data Type Conversion2/1 -> Assign Joint Trajectory Point/3, Assign Joint Trajectory Point/2
  dq/1 -> Assignment1/2
  Blank Message2/1 -> Assign Joint Trajectory Point/1
  vel/1 -> Assignment1/1
  Assignment1/1 -> Assign Joint Trajectory Point/5
  time/1 -> Add/1, Rounding Function/1
  Rounding Function/1 -> Assign Joint Trajectory Point/6, Add/2  "decimalPart"
  Add/1 -> Gain/1  "fractionalPart"

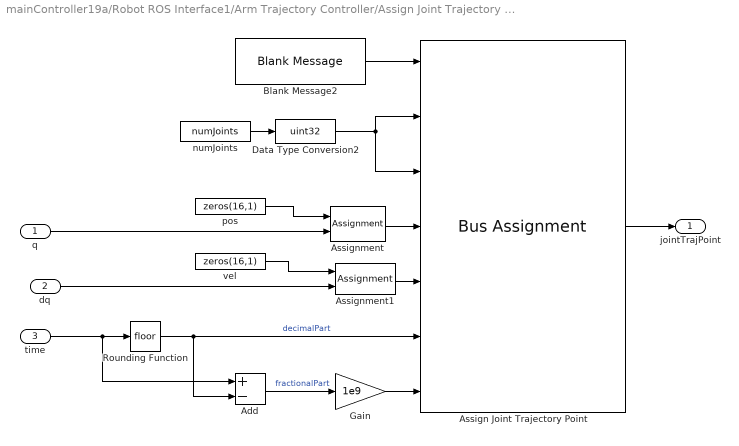
== system mainController19a/Robot ROS Interface1/Arm Trajectory Controller/Assign Joint Trajectory Point3 ==
  q : Inport
  dq : Inport  Port=2
  time : Inport  Port=3
  Add : Sum  Inputs=+-
  Assign Joint Trajectory Point : BusAssignment  AssignedSignals=Positions_SL_Info.CurrentLength,Velocities_SL_Info.CurrentLength,Positions,Velocities,TimeFromStart.Sec,TimeFromStart.Nsec
  Assignment : Assignment  DiagnosticForDimensions=Warning  IndexOptions=Index vector (dialog)  Indices=1:numJoints  OutputSizes=1
  Assignment1 : Assignment  DiagnosticForDimensions=Warning  IndexOptions=Index vector (dialog)  Indices=1:numJoints  OutputSizes=1
  Blank Message2 : robotlib/Blank Message  messageClass=Message  entityType=trajectory_msgs/JointTrajectoryPoint  messageType=trajectory_msgs/JointTrajectoryPoint  SampleTime=-1
      settings: SourceProductBaseCode=RO
  Data Type Conversion2 : DataTypeConversion  OutDataTypeStr=uint32
  Gain : Gain  Gain=1e9
  Rounding Function : Rounding
  numJoints : Constant  Value=numJoints
  pos : Constant  Value=zeros(16,1)
  vel : Constant  Value=zeros(16,1)
  jointTrajPoint : Outport
  wires:
  Add/1 -> Gain/1  "fractionalPart"
  Rounding Function/1 -> Add/2, Assign Joint Trajectory Point/6  "decimalPart"
  time/1 -> Rounding Function/1, Add/1
  Assignment1/1 -> Assign Joint Trajectory Point/5
  vel/1 -> Assignment1/1
  Blank Message2/1 -> Assign Joint Trajectory Point/1
  dq/1 -> Assignment1/2
  Data Type Conversion2/1 -> Assign Joint Trajectory Point/2, Assign Joint Trajectory Point/3
  numJoints/1 -> Data Type Conversion2/1
  q/1 -> Assignment/2
  Gain/1 -> Assign Joint Trajectory Point/7
  pos/1 -> Assignment/1
  Assign Joint Trajectory Point/1 -> jointTrajPoint/1
  Assignment/1 -> Assign Joint Trajectory Point/4

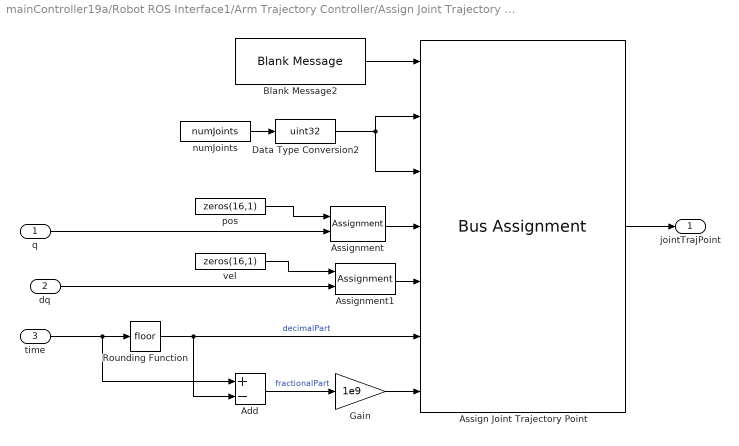
== system mainController19a/Robot ROS Interface1/Arm Trajectory Controller/Assign Joint Trajectory Point4 ==
  q : Inport
  dq : Inport  Port=2
  time : Inport  Port=3
  Add : Sum  Inputs=+-
  Assign Joint Trajectory Point : BusAssignment  AssignedSignals=Positions_SL_Info.CurrentLength,Velocities_SL_Info.CurrentLength,Positions,Velocities,TimeFromStart.Sec,TimeFromStart.Nsec
  Assignment : Assignment  DiagnosticForDimensions=Warning  IndexOptions=Index vector (dialog)  Indices=1:numJoints  OutputSizes=1
  Assignment1 : Assignment  DiagnosticForDimensions=Warning  IndexOptions=Index vector (dialog)  Indices=1:numJoints  OutputSizes=1
  Blank Message2 : robotlib/Blank Message  messageClass=Message  entityType=trajectory_msgs/JointTrajectoryPoint  messageType=trajectory_msgs/JointTrajectoryPoint  SampleTime=-1
      settings: SourceProductBaseCode=RO
  Data Type Conversion2 : DataTypeConversion  OutDataTypeStr=uint32
  Gain : Gain  Gain=1e9
  Rounding Function : Rounding
  numJoints : Constant  Value=numJoints
  pos : Constant  Value=zeros(16,1)
  vel : Constant  Value=zeros(16,1)
  jointTrajPoint : Outport
  wires:
  Assignment/1 -> Assign Joint Trajectory Point/4
  Assign Joint Trajectory Point/1 -> jointTrajPoint/1
  pos/1 -> Assignment/1
  Gain/1 -> Assign Joint Trajectory Point/7
  q/1 -> Assignment/2
  numJoints/1 -> Data Type Conversion2/1
  Data Type Conversion2/1 -> Assign Joint Trajectory Point/3, Assign Joint Trajectory Point/2
  dq/1 -> Assignment1/2
  Blank Message2/1 -> Assign Joint Trajectory Point/1
  vel/1 -> Assignment1/1
  Assignment1/1 -> Assign Joint Trajectory Point/5
  time/1 -> Add/1, Rounding Function/1
  Rounding Function/1 -> Assign Joint Trajectory Point/6, Add/2  "decimalPart"
  Add/1 -> Gain/1  "fractionalPart"

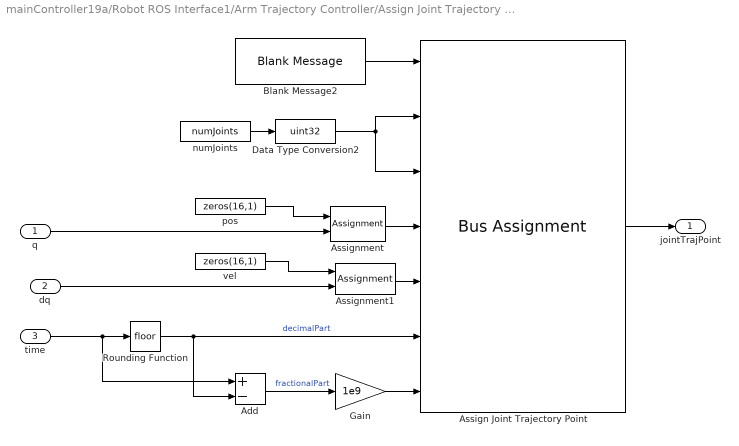
== system mainController19a/Robot ROS Interface1/Arm Trajectory Controller/Assign Joint Trajectory Point5 ==
  q : Inport
  dq : Inport  Port=2
  time : Inport  Port=3
  Add : Sum  Inputs=+-
  Assign Joint Trajectory Point : BusAssignment  AssignedSignals=Positions_SL_Info.CurrentLength,Velocities_SL_Info.CurrentLength,Positions,Velocities,TimeFromStart.Sec,TimeFromStart.Nsec
  Assignment : Assignment  DiagnosticForDimensions=Warning  IndexOptions=Index vector (dialog)  Indices=1:numJoints  OutputSizes=1
  Assignment1 : Assignment  DiagnosticForDimensions=Warning  IndexOptions=Index vector (dialog)  Indices=1:numJoints  OutputSizes=1
  Blank Message2 : robotlib/Blank Message  messageClass=Message  entityType=trajectory_msgs/JointTrajectoryPoint  messageType=trajectory_msgs/JointTrajectoryPoint  SampleTime=-1
      settings: SourceProductBaseCode=RO
  Data Type Conversion2 : DataTypeConversion  OutDataTypeStr=uint32
  Gain : Gain  Gain=1e9
  Rounding Function : Rounding
  numJoints : Constant  Value=numJoints
  pos : Constant  Value=zeros(16,1)
  vel : Constant  Value=zeros(16,1)
  jointTrajPoint : Outport
  wires:
  Add/1 -> Gain/1  "fractionalPart"
  Rounding Function/1 -> Add/2, Assign Joint Trajectory Point/6  "decimalPart"
  time/1 -> Rounding Function/1, Add/1
  Assignment1/1 -> Assign Joint Trajectory Point/5
  vel/1 -> Assignment1/1
  Blank Message2/1 -> Assign Joint Trajectory Point/1
  dq/1 -> Assignment1/2
  Data Type Conversion2/1 -> Assign Joint Trajectory Point/2, Assign Joint Trajectory Point/3
  numJoints/1 -> Data Type Conversion2/1
  q/1 -> Assignment/2
  Gain/1 -> Assign Joint Trajectory Point/7
  pos/1 -> Assignment/1
  Assign Joint Trajectory Point/1 -> jointTrajPoint/1
  Assignment/1 -> Assign Joint Trajectory Point/4

== system mainController19a/Robot ROS Interface1/Arm Trajectory Controller/Split Matrix ==
  qMatrix : Inport
  dqMatrix : Inport  Port=2
  tVector : Inport  Port=3
  index : Inport  Port=4
  Selector : Selector  NumberOfDimensions=2  InputPortWidth=3  IndexOptions=Select all,Index vector (port)  Indices=[1 3],1  OutputSizes=1,1
  Selector1 : Selector  IndexOptions=Index vector (port)  Indices=[1 3]  OutputSizes=1
  Selector5 : Selector  NumberOfDimensions=2  InputPortWidth=3  IndexOptions=Select all,Index vector (port)  Indices=[1 3],1  OutputSizes=1,1
  q : Outport
  dq : Outport  Port=2
  t : Outport  Port=3
  wires:
  Selector/1 -> q/1
  index/1 -> Selector/2, Selector5/2, Selector1/2
  qMatrix/1 -> Selector/1
  tVector/1 -> Selector1/1
  Selector1/1 -> t/1
  dqMatrix/1 -> Selector5/1
  Selector5/1 -> dq/1

== system mainController19a/Robot ROS Interface1/Arm Trajectory Controller/Split Matrix1 ==
  qMatrix : Inport
  dqMatrix : Inport  Port=2
  tVector : Inport  Port=3
  index : Inport  Port=4
  Selector : Selector  NumberOfDimensions=2  InputPortWidth=3  IndexOptions=Select all,Index vector (port)  Indices=[1 3],1  OutputSizes=1,1
  Selector1 : Selector  IndexOptions=Index vector (port)  Indices=[1 3]  OutputSizes=1
  Selector5 : Selector  NumberOfDimensions=2  InputPortWidth=3  IndexOptions=Select all,Index vector (port)  Indices=[1 3],1  OutputSizes=1,1
  q : Outport
  dq : Outport  Port=2
  t : Outport  Port=3
  wires:
  Selector5/1 -> dq/1
  dqMatrix/1 -> Selector5/1
  Selector1/1 -> t/1
  tVector/1 -> Selector1/1
  qMatrix/1 -> Selector/1
  index/1 -> Selector1/2, Selector5/2, Selector/2
  Selector/1 -> q/1

== system mainController19a/Robot ROS Interface1/Arm Trajectory Controller/Split Matrix2 ==
  qMatrix : Inport
  dqMatrix : Inport  Port=2
  tVector : Inport  Port=3
  index : Inport  Port=4
  Selector : Selector  NumberOfDimensions=2  InputPortWidth=3  IndexOptions=Select all,Index vector (port)  Indices=[1 3],1  OutputSizes=1,1
  Selector1 : Selector  IndexOptions=Index vector (port)  Indices=[1 3]  OutputSizes=1
  Selector5 : Selector  NumberOfDimensions=2  InputPortWidth=3  IndexOptions=Select all,Index vector (port)  Indices=[1 3],1  OutputSizes=1,1
  q : Outport
  dq : Outport  Port=2
  t : Outport  Port=3
  wires:
  Selector/1 -> q/1
  index/1 -> Selector/2, Selector5/2, Selector1/2
  qMatrix/1 -> Selector/1
  tVector/1 -> Selector1/1
  Selector1/1 -> t/1
  dqMatrix/1 -> Selector5/1
  Selector5/1 -> dq/1

== system mainController19a/Robot ROS Interface1/Arm Trajectory Controller/Split Matrix3 ==
  qMatrix : Inport
  dqMatrix : Inport  Port=2
  tVector : Inport  Port=3
  index : Inport  Port=4
  Selector : Selector  NumberOfDimensions=2  InputPortWidth=3  IndexOptions=Select all,Index vector (port)  Indices=[1 3],1  OutputSizes=1,1
  Selector1 : Selector  IndexOptions=Index vector (port)  Indices=[1 3]  OutputSizes=1
  Selector5 : Selector  NumberOfDimensions=2  InputPortWidth=3  IndexOptions=Select all,Index vector (port)  Indices=[1 3],1  OutputSizes=1,1
  q : Outport
  dq : Outport  Port=2
  t : Outport  Port=3
  wires:
  Selector5/1 -> dq/1
  dqMatrix/1 -> Selector5/1
  Selector1/1 -> t/1
  tVector/1 -> Selector1/1
  qMatrix/1 -> Selector/1
  index/1 -> Selector1/2, Selector5/2, Selector/2
  Selector/1 -> q/1

== system mainController19a/Robot ROS Interface1/Arm Trajectory Controller/Split Matrix4 ==
  qMatrix : Inport
  dqMatrix : Inport  Port=2
  tVector : Inport  Port=3
  index : Inport  Port=4
  Selector : Selector  NumberOfDimensions=2  InputPortWidth=3  IndexOptions=Select all,Index vector (port)  Indices=[1 3],1  OutputSizes=1,1
  Selector1 : Selector  IndexOptions=Index vector (port)  Indices=[1 3]  OutputSizes=1
  Selector5 : Selector  NumberOfDimensions=2  InputPortWidth=3  IndexOptions=Select all,Index vector (port)  Indices=[1 3],1  OutputSizes=1,1
  q : Outport
  dq : Outport  Port=2
  t : Outport  Port=3
  wires:
  Selector/1 -> q/1
  index/1 -> Selector/2, Selector5/2, Selector1/2
  qMatrix/1 -> Selector/1
  tVector/1 -> Selector1/1
  Selector1/1 -> t/1
  dqMatrix/1 -> Selector5/1
  Selector5/1 -> dq/1

== system mainController19a/Robot ROS Interface1/Arm Trajectory Controller/Split Matrix5 ==
  qMatrix : Inport
  dqMatrix : Inport  Port=2
  tVector : Inport  Port=3
  index : Inport  Port=4
  Selector : Selector  NumberOfDimensions=2  InputPortWidth=3  IndexOptions=Select all,Index vector (port)  Indices=[1 3],1  OutputSizes=1,1
  Selector1 : Selector  IndexOptions=Index vector (port)  Indices=[1 3]  OutputSizes=1
  Selector5 : Selector  NumberOfDimensions=2  InputPortWidth=3  IndexOptions=Select all,Index vector (port)  Indices=[1 3],1  OutputSizes=1,1
  q : Outport
  dq : Outport  Port=2
  t : Outport  Port=3
  wires:
  Selector5/1 -> dq/1
  dqMatrix/1 -> Selector5/1
  Selector1/1 -> t/1
  tVector/1 -> Selector1/1
  qMatrix/1 -> Selector/1
  index/1 -> Selector1/2, Selector5/2, Selector/2
  Selector/1 -> q/1

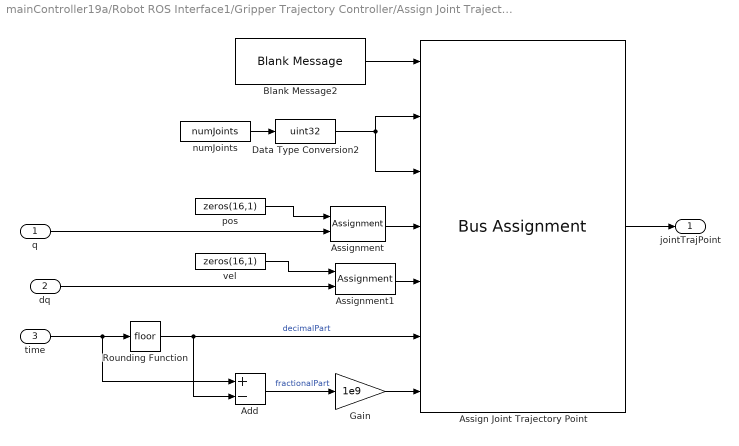
== system mainController19a/Robot ROS Interface1/Gripper Trajectory Controller/Assign Joint Trajectory Point ==
  q : Inport
  dq : Inport  Port=2
  time : Inport  Port=3
  Add : Sum  Inputs=+-
  Assign Joint Trajectory Point : BusAssignment  AssignedSignals=Positions_SL_Info.CurrentLength,Velocities_SL_Info.CurrentLength,Positions,Velocities,TimeFromStart.Sec,TimeFromStart.Nsec
  Assignment : Assignment  DiagnosticForDimensions=Warning  IndexOptions=Index vector (dialog)  Indices=1:numJoints  OutputSizes=1
  Assignment1 : Assignment  DiagnosticForDimensions=Warning  IndexOptions=Index vector (dialog)  Indices=1:numJoints  OutputSizes=1
  Blank Message2 : robotlib/Blank Message  messageClass=Message  entityType=trajectory_msgs/JointTrajectoryPoint  messageType=trajectory_msgs/JointTrajectoryPoint  SampleTime=-1
      settings: SourceProductBaseCode=RO
  Data Type Conversion2 : DataTypeConversion  OutDataTypeStr=uint32
  Gain : Gain  Gain=1e9
  Rounding Function : Rounding
  numJoints : Constant  Value=numJoints
  pos : Constant  Value=zeros(16,1)
  vel : Constant  Value=zeros(16,1)
  jointTrajPoint : Outport
  wires:
  Add/1 -> Gain/1  "fractionalPart"
  Rounding Function/1 -> Add/2, Assign Joint Trajectory Point/6  "decimalPart"
  time/1 -> Rounding Function/1, Add/1
  Assignment1/1 -> Assign Joint Trajectory Point/5
  vel/1 -> Assignment1/1
  Blank Message2/1 -> Assign Joint Trajectory Point/1
  dq/1 -> Assignment1/2
  Data Type Conversion2/1 -> Assign Joint Trajectory Point/2, Assign Joint Trajectory Point/3
  numJoints/1 -> Data Type Conversion2/1
  q/1 -> Assignment/2
  Gain/1 -> Assign Joint Trajectory Point/7
  pos/1 -> Assignment/1
  Assign Joint Trajectory Point/1 -> jointTrajPoint/1
  Assignment/1 -> Assign Joint Trajectory Point/4

== system mainController19a/Robot ROS Interface1/Kinect Data/Extract Point Cloud Data ==
  pcloudMsg : Inport
  Enable : EnablePort  PropagateVarSize=During execution
  Display : Display
  Read Point Cloud : robotlib/Read Point Cloud  MaximumPointCloudSize=[424, 512]  PreserveStructure=on  ShowRGBOutput=on  ShowIntensityOutput=off  ShowErrorCodeOutput=on  VariableSizeOutputs=off
      settings: SourceProductName=Robotics System Toolbox  SourceProductBaseCode=RO
  RGB : Outport
  XYZ : Outport  Port=2
  wires:
  Read Point Cloud/3 -> Display/1
  pcloudMsg/1 -> Read Point Cloud/1
  Read Point Cloud/2 -> RGB/1
  Read Point Cloud/1 -> XYZ/1

== system mainController19a/Robot ROS Interface1/Robot State/Get Finger Positions ==
  msg : Inport
  Enable : EnablePort
  Bus Selector : BusSelector  OutputSignals=Actual.Positions,Actual.Positions_SL_Info.CurrentLength
  Constant : Constant  Value=numJoints
  Data Type Conversion : DataTypeConversion  OutDataTypeStr=uint32
  Relational Operator : RelationalOperator  Operator===  OutDataTypeStr=boolean  RndMeth=Simplest
  Selector : Selector  InputPortWidth=16  IndexOptions=Index vector (dialog)  Indices=[1:numJoints]  OutputSizes=1
  gripperAct : Outport  InitialOutput=-1000*ones(numJoints,1)
  isValid : Outport  Port=2  InitialOutput=[0]
  wires:
  Relational Operator/1 -> isValid/1
  Data Type Conversion/1 -> Relational Operator/2
  Constant/1 -> Data Type Conversion/1
  Selector/1 -> gripperAct/1
  Bus Selector/2 -> Relational Operator/1  "<CurrentLength>"
  Bus Selector/1 -> Selector/1  "<Positions>"
  msg/1 -> Bus Selector/1

== system mainController19a/Robot ROS Interface1/Robot State/Get Joint Positions ==
  msg : Inport
  Enable : EnablePort
  Bus Selector : BusSelector  OutputSignals=Actual.Positions,Actual.Positions_SL_Info.CurrentLength
  Constant : Constant  Value=numJoints
  Data Type Conversion : DataTypeConversion  OutDataTypeStr=uint32
  Relational Operator : RelationalOperator  Operator===  OutDataTypeStr=boolean  RndMeth=Simplest
  Selector : Selector  InputPortWidth=16  IndexOptions=Index vector (dialog)  Indices=[1:numJoints]  OutputSizes=1
  qAct : Outport  InitialOutput=-1000*ones(numJoints,1)
  isValid : Outport  Port=2  InitialOutput=[0]
  wires:
  msg/1 -> Bus Selector/1
  Bus Selector/1 -> Selector/1  "<Positions>"
  Bus Selector/2 -> Relational Operator/1  "<CurrentLength>"
  Selector/1 -> qAct/1
  Constant/1 -> Data Type Conversion/1
  Data Type Conversion/1 -> Relational Operator/2
  Relational Operator/1 -> isValid/1

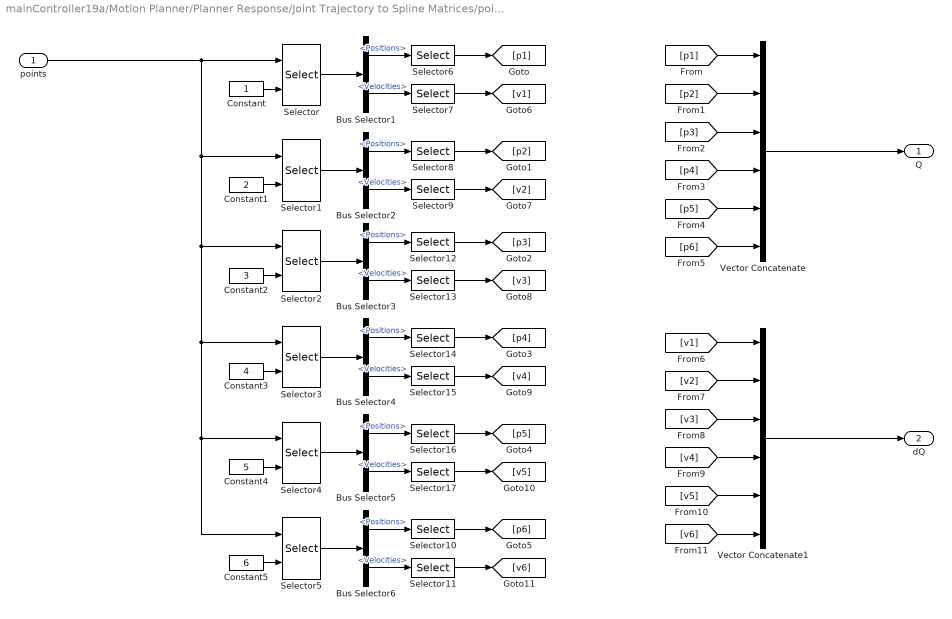
== system mainController19a/Motion Planner/Planner Response/Joint Trajectory to Spline Matrices/pointsToSplineWithBlocks ==
  points : Inport
  Bus Selector{1..6} (6 alike) : BusSelector  OutputSignals=Positions,Velocities
  Constant : Constant
  Constant1 : Constant  Value=2
  Constant2 : Constant  Value=3
  Constant3 : Constant  Value=4
  Constant4 : Constant  Value=5
  Constant5 : Constant  Value=6
  Selector{,1..5} (6 alike) : Selector  InputPortWidth=16  IndexOptions=Index vector (port)  Indices=[1]  OutputSizes=1
  Selector{6..17} (12 alike) : Selector  IndexOptions=Index vector (dialog)  Indices=[1:numJoints]  OutputSizes=1
  Vector Concatenate : Concatenate  NumInputs=6  Mode=Multidimensional array  ConcatenateDimension=2
  Vector Concatenate1 : Concatenate  NumInputs=6  Mode=Multidimensional array  ConcatenateDimension=2
  Q : Outport
  dQ : Outport  Port=2
  wires:
  [v4] -> Vector Concatenate1/4
  Constant1/1 -> Selector1/2
  Bus Selector5/1 -> Selector16/1  "<Positions>"
  Constant5/1 -> Selector5/2
  Bus Selector3/1 -> Selector12/1  "<Positions>"
  Selector4/1 -> Bus Selector5/1
  Vector Concatenate/1 -> Q/1
  Bus Selector3/2 -> Selector13/1  "<Velocities>"
  Bus Selector4/2 -> Selector15/1  "<Velocities>"
  Bus Selector1/1 -> Selector6/1  "<Positions>"
  Bus Selector2/2 -> Selector9/1  "<Velocities>"
  Selector/1 -> Bus Selector1/1
  points/1 -> Selector1/1, Selector2/1, Selector3/1, Selector4/1, Selector5/1, Selector/1
  Bus Selector6/2 -> Selector11/1  "<Velocities>"
  Selector1/1 -> Bus Selector2/1
  Constant/1 -> Selector/2
  Bus Selector5/2 -> Selector17/1  "<Velocities>"
  Selector3/1 -> Bus Selector4/1
  Selector5/1 -> Bus Selector6/1
  Selector2/1 -> Bus Selector3/1
  Bus Selector4/1 -> Selector14/1  "<Positions>"
  Bus Selector2/1 -> Selector8/1  "<Positions>"
  Constant3/1 -> Selector3/2
  Constant2/1 -> Selector2/2
  Bus Selector1/2 -> Selector7/1  "<Velocities>"
  Constant4/1 -> Selector4/2
  Bus Selector6/1 -> Selector10/1  "<Positions>"
  Selector6/1 -> [p1]
  Selector17/1 -> [v5]
  [v5] -> Vector Concatenate1/5
  Selector12/1 -> [p3]
  Selector8/1 -> [p2]
  Selector15/1 -> [v4]
  Selector14/1 -> [p4]
  Vector Concatenate1/1 -> dQ/1
  [v6] -> Vector Concatenate1/6
  [p4] -> Vector Concatenate/4
  [v3] -> Vector Concatenate1/3
  Selector16/1 -> [p5]
  [p3] -> Vector Concatenate/3
  Selector9/1 -> [v2]
  [p6] -> Vector Concatenate/6
  Selector13/1 -> [v3]
  [p1] -> Vector Concatenate/1
  Selector7/1 -> [v1]
  [v1] -> Vector Concatenate1/1
  [p2] -> Vector Concatenate/2
  [v2] -> Vector Concatenate1/2
  Selector11/1 -> [v6]
  [p5] -> Vector Concatenate/5
  Selector10/1 -> [p6]
